simulink model "PI"  (R2025b)
settings: Solver=VariableStepAuto  StartTime=0.0  StopTime=2  RelTol=1e-3
InitFcn:
  | cd("C:\Github\Tesis\src\matlab\Simulaciones Controladores\BP");
  | load("modelo.mat");
StartFcn:
  | load("modelo.mat");
undefined symbols (not defined in the file or in its folder): dspblkCoreblockFVToolHelper, gcbh, linsys1
libraries: dspswit3 x1, slpidlib x1
settings Model: Creator=elias  LastModifiedBy=elias

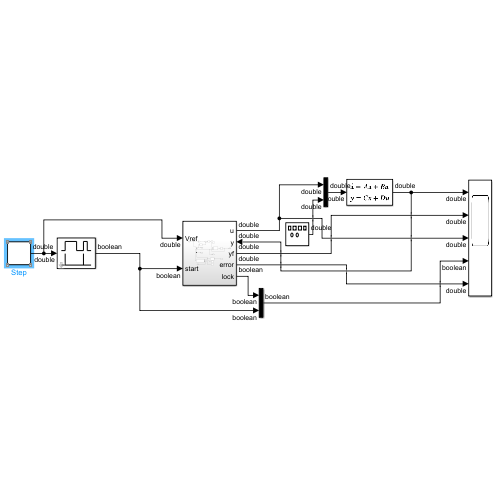
[thumbnail: Simulink's stored preview of the top-level diagram]
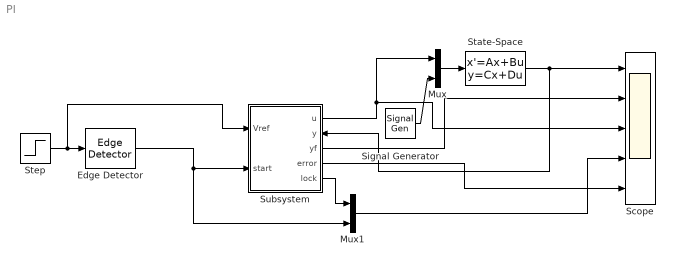
== system PI ==
  Edge Detector : dspswit3/Edge Detector
  Mux : Mux  Inputs=2
  Mux1 : Mux  Inputs=2
  Scope : Scope  NumInputPorts=5
      settings: ActiveDisplayYMinimum=-0.61485747802995938  ActiveDisplayYMaximum=4.5337977527076365
  Signal Generator : SignalGenerator  WaveForm=random  Amplitude=1e-3  Frequency=3000
  State-Space : StateSpace  A=linsys1.A  B=linsys1.B  C=linsys1.C  D=linsys1.D  InitialCondition=0
  Step : Step  SampleTime=1/3000
  Subsystem : Subsystem
      settings: PortSchema="{\"entries\":[{\"content\":{\"sides\":[{\"content\":{\"connectorIds\":[\"In1\",\"In2\"]},\"type\":\"ConnectorPlacement.EquallySpacedRectSide\",\"uuid\":\"f954b099-4229-4382-8854-0a3de070809c\"},{\"content\":{\"connectorIds\":[\"Out1\",\"In3\",\"Out2\",\"Out3\",\"Out4\"],\"side\":\"RIGHT\"},\"type\":\"ConnectorPlacement.EquallySpacedRectSide\",\"uuid\":\"a68b1462-0060-4c69-b688-538e441c0c98\"},{\"content\":{\"side\":\"TOP\"},\"type\":\"ConnectorPlacement.EquallySpacedRectSide\",\"uuid\":\"04b4dfef-d756-429a-8752-10270254ecef\"}]},\"type\":\"ConnectorPlacement.EquallySpacedConnector\",\"uuid\":\"b45df344-c4ba-4f65-9a35-6e5f0bedc7fa\"}],\"packageUris\":[\"http://schema.mathworks.com/mf0/Connector/R2020b\"],\"version\":\"1.0\"}"
  wires:
  Mux/1 -> State-Space/1
  Subsystem/1(u) -> Scope/3, Mux/1
  Step/1 -> Subsystem/1(Vref), Edge Detector/1
  State-Space/1 -> Scope/1, Subsystem/3(y)
  Signal Generator/1 -> Mux/2
  Subsystem/2(yf) -> Scope/2
  Subsystem/4(lock) -> Mux1/1
  Edge Detector/1 -> Mux1/2, Subsystem/2(start)
  Mux1/1 -> Scope/4
  Subsystem/3(error) -> Scope/5

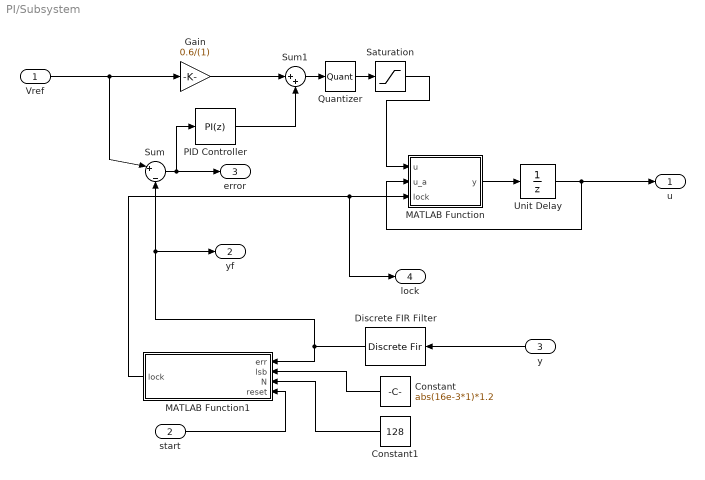
== system PI/Subsystem ==
  Vref : Inport
  start : Inport  Port=2
  y : Inport  Port=3
  Constant : Constant  Value=abs(16e-3*1)*1.2  SampleTime=1/3000
  Constant1 : Constant  Value=128
  Discrete FIR Filter : DiscreteFir  LoadFcn=dspblkCoreblockFVToolHelper(gcbh,'load');  Coefficients=fir1(127, 0.1/1500, hamming(127+1))
      settings: CopyFcn=dspblkCoreblockFVToolHelper(gcbh,'copy');  DeleteFcn=dspblkCoreblockFVToolHelper(gcbh,'close');  ModelCloseFcn=dspblkCoreblockFVToolHelper(gcbh,'close');  PreSaveFcn=dspblkCoreblockFVToolHelper(gcbh,'presave');  PostSaveFcn=dspblkCoreblockFVToolHelper(gcbh,'postsave');  CloseFcn=dspblkCoreblockFVToolHelper(gcbh,'close');
  Gain : Gain  Gain=0.6/(1)
  MATLAB Function : MATLAB Function  TreatAsAtomicUnit=on
  MATLAB Function1 : MATLAB Function  TreatAsAtomicUnit=on
  PID Controller : slpidlib/PID Controller  Controller=PI  Form=Parallel  TimeDomain=Discrete-time  UseExternalTs=off  SampleTime=-1  IntegratorMethod=Forward Euler  FilterMethod=Forward Euler  ControllerParametersSource=internal  P=-1e-3  I=-300e-6  UseKiTs=on  D=0  UseExternalDerivativeSource=off  N=100  UseFilter=on  TunerSelectOption=Transfer Function Based (PID Tuner App)  InitialConditionSource=internal  InitialConditionForIntegrator=0  InitialConditionForFilter=0  DifferentiatorICPrevScaledInput=0  ExternalReset=none  TrackingMode=off  Kt=1  LimitOutput=on  SatLimitsSource=internal  UpperSaturationLimit=4.08  LowerSaturationLimit=0  LinearizeAsGain=off  AntiWindupMode=clamping  Kb=1  LimitIntegrator=on  UpperIntegratorSaturationLimit=4.08  LowerIntegratorSaturationLimit=0  POutMin=[]  POutMax=[]  IOutMin=[]  IOutMax=[]  DOutMin=[]  DOutMax=[]  NOutMin=[]  NOutMax=[]  SumOutMin=[]  SumOutMax=[]  SaturationOutMin=[]  SaturationOutMax=[]  PParamMin=[]  PParamMax=[]  IParamMin=[]  IParamMax=[]  DParamMin=[]  DParamMax=[]  NParamMin=[]  NParamMax=[]  KbParamMin=[]  KbParamMax=[]  KtParamMin=[]  KtParamMax=[]  KbOutMin=[]  KbOutMax=[]  KtOutMin=[]  KtOutMax=[]  IntegratorOutMin=[]  IntegratorOutMax=[]  FilterOutMin=[]  FilterOutMax=[]  SumI1OutMin=[]  SumI1OutMax=[]  SumI2OutMin=[]  SumI2OutMax=[]  SumI3OutMin=[]  SumI3OutMax=[]  SumI4OutMin=[]  SumI4OutMax=[]  SumDOutMin=[]  SumDOutMax=[]  DifferentiatorOutMin=[]  DifferentiatorOutMax=[]  FilterDiffOutCoefMin=[]  FilterDiffOutCoefMax=[]  ReciprocalOutMin=[]  ReciprocalOutMax=[]  SumDenOutMin=[]  SumDenOutMax=[]  SumNumOutMin=[]  SumNumOutMax=[]  DivideOutMin=[]  DivideOutMax=[]  UdiffTsProdOutMin=[]  UdiffTsProdOutMax=[]  NTsProdOutMin=[]  NTsProdOutMax=[]  UintegralTsProdOutMin=[]  UintegralTsProdOutMax=[]  UngainTsProdOutMin=[]  UngainTsProdOutMax=[]  ClampingZeroOutDataTypeStr=Inherit: Inherit via back propagation  ClampingZeroOutMin=[]  ClampingZeroOutMax=[]  FilterDenConstantOutDataTypeStr=Inherit: Inherit via back propagation  FilterDenConstantOutMin=[]  FilterDenConstantOutMax=[]  PCopyOutDataTypeStr=Inherit: Inherit via back propagation  PCopyOutMin=[]  PCopyOutMax=[]  NCopyOutDataTypeStr=Inherit: Inherit via back propagation  NCopyOutMin=[]  NCopyOutMax=[]  IntegratorContinuousStateAttributes=''  IntegratorStateMustResolveToSignalObject=off  IntegratorRTWStateStorageClass=Auto  FilterContinuousStateAttributes=''  FilterStateMustResolveToSignalObject=off  FilterRTWStateStorageClass=Auto  ParallelPVariant=InternalParameters  IdealPVariant=Disabled  IVariant=InternalParameters  DVariant=Disabled  IntegratorVariant=Discrete  SatVariant=Enabled  AWVariant=DiscClampingParallel  PCopyVariant=Disabled  TRVariant=Disabled  FdbkBlocksVariant=Forward  IdealPFdbkVariant=Disabled  SatFdbkVariant=Disabled  DerivativeFilterVariant=Disabled  NVariant=Disabled  NCopyVariant=Disabled_SignalSpec  FilterICVariant=Disabled  IntegratorICVariant=InternalICs  ExternalResetVariant=Disabled  TRSumVariant=Passthrough  SumFdbkVariant=Disabled  SumVariant=Sum_PI  TsampFilterVariant=InternalTs  TsampNgainVariant=Passthrough  TsampIntegralVariant=Disabled_SignalSpec  ExternalSaturationOutDataTypeStr=Inherit: Same as second input  DerivativeSourceVariant=Disabled  PreIntVariant=InternalPreInt
  Quantizer : Quantizer  QuantizationInterval=16e-3
  Saturation : Saturate  UpperLimit=2.5  LowerLimit=-2.5
  Sum : Sum  Inputs=|+|-
  Sum1 : Sum  Inputs=|++
  Unit Delay : UnitDelay  SampleTime=-1  HasFrameUpgradeWarning=on
  u : Outport
  yf : Outport  Port=2
  error : Outport  Port=3
  lock : Outport  Port=4
  wires:
  Sum1/1 -> Quantizer/1
  Unit Delay/1 -> u/1, MATLAB Function/2(u_a)
  Discrete FIR Filter/1 -> yf/1, Sum/2, MATLAB Function1/1(err)
  Gain/1 -> Sum1/1
  Vref/1 -> Sum/1, Gain/1
  Saturation/1 -> MATLAB Function/1(u)
  y/1 -> Discrete FIR Filter/1
  MATLAB Function1/1(lock) -> lock/1, MATLAB Function/3(lock)
  PID Controller/1 -> Sum1/2
  Constant/1 -> MATLAB Function1/2(lsb)
  start/1 -> MATLAB Function1/4(reset)
  Sum/1 -> error/1, PID Controller/1
  MATLAB Function/1(y) -> Unit Delay/1
  Constant1/1 -> MATLAB Function1/3(N)
  Quantizer/1 -> Saturation/1

== matlab function PI/Subsystem/MATLAB Function1 ==
  data: err input; lsb input; N input; reset input; lock output
function lock = detect_lock(err, lsb, N, reset)
%#codegen

persistent buf idx count locked

if isempty(buf)
    buf = zeros(1, N);
    idx = 1;
    count = 0;
    locked = false;
end

if reset
    buf(:) = 0;
    idx = 1;
    count = 0;
    locked = false;
    lock = false;
    return;
end

buf(idx) = err;

idx = idx + 1;
if idx > N
    idx = 1;
end

if count < N
    count = count + 1;
end

if count < N
    lock = false;
    return;
end

err_span = max(buf) - min(buf);

lock_threshold   = lsb;
unlock_threshold = 2*lsb;

if ~locked
    if err_span <= lock_threshold
        locked = true;
    end
else
    if err_span > unlock_threshold
        locked = false;
    end
end

lock = locked;

== matlab function PI/Subsystem/MATLAB Function ==
  data: u input; u_a input; lock input; y output
function y = fcn(u, u_a,lock)
    if lock == 1
        y = u_a;
    else
        y = u;
    end
end
